simulink model "Subsistema_Fisico_No_Lineal"  (R2024b)
settings: Solver=VariableStepAuto  StartTime=0.0  StopTime=10.0  RelTol=1e-3
values from neighbouring files (symbols this model uses):
  alpha_cu = 3.9 *10^-3    (= 0.0039)    [parametros.m]
  b_eq = b_m + (1/r^2) * b_l    (= 2.19444444444e-05)    [parametros.m]
  C_ts = 0.818    [parametros.m]
  g = 9.80665    [parametros.m]
  J_eq = J_m + (1/r^2) * J_l    (= 4.58263888889e-05)    [parametros.m]
  k_l = m * l_cm + m_l* l_l    (= 1)    [parametros.m]
  L_d = 6.6 * 10^-3    (= 0.0066)    [parametros.m]
  L_ls = 0.8 * 10^-3    (= 0.0008)    [parametros.m]
  L_q = 5.8 * 10^-3    (= 0.0058)    [parametros.m]
  lambda_m = 0.016    [parametros.m]
  P_p = 3    [parametros.m]
  r = 120    [parametros.m]
  R_s_40 = 1.02    [parametros.m]
  R_ts_amb = 146.7    [parametros.m]
  Temp_s_ref = 20    [parametros.m]
settings Model: Creator=nsorr  LastModifiedBy=nsorr

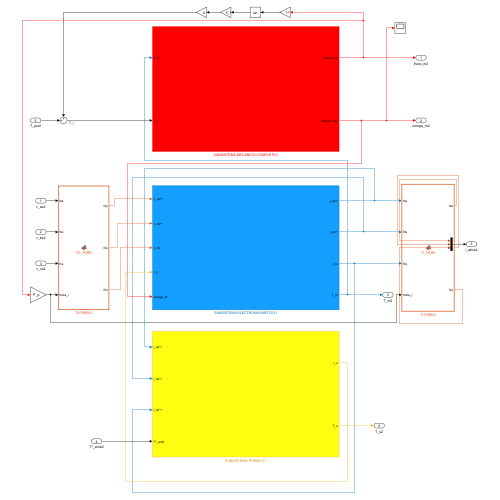
[thumbnail: Simulink's stored preview of the top-level diagram]
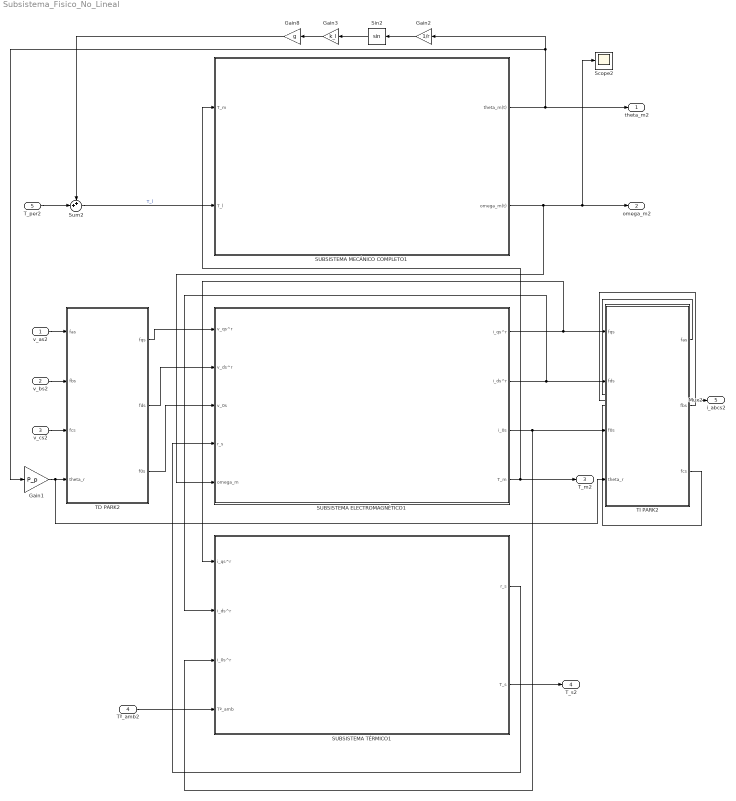
== system Subsistema_Fisico_No_Lineal ==
  v_as2 : Inport
  v_bs2 : Inport  Port=2
  v_cs2 : Inport  Port=3
  Tº_amb2 : Inport  Port=4
  T_per2 : Inport  Port=5
  Gain1 : Gain  Gain=P_p
  Gain2 : Gain  Gain=1/r
  Gain3 : Gain  Gain=k_l
  Gain8 : Gain  Gain=g
  Mux2 : Mux  Inputs=3
  SUBSISTEMA ELECTROMAGNÉTICO1 : Subsystem
  SUBSISTEMA MECÁNICO COMPLETO1 : Subsystem
  SUBSISTEMA TÉRMICO1 : Subsystem
  Scope2 : Scope
  Sin2 : Trigonometry
  Sum2 : Sum  Inputs=++|
  TD PARK2 : MATLAB Function  TreatAsAtomicUnit=on
  TI PARK2 : MATLAB Function  TreatAsAtomicUnit=on
  theta_m2 : Outport
  omega_m2 : Outport  Port=2
  T_m2 : Outport  Port=3
  T_s2 : Outport  Port=4
  i_abcs2 : Outport  Port=5
  wires:
  Sin2/1 -> Gain3/1
  Mux2/1 -> i_abcs2/1
  Gain3/1 -> Gain8/1
  TI PARK2/1(fas) -> Mux2/1
  v_cs2/1 -> TD PARK2/3(fcs)
  SUBSISTEMA ELECTROMAGNÉTICO1/2(i_ds^r) -> SUBSISTEMA TÉRMICO1/2(i_ds^r), TI PARK2/2(fds)
  Gain1/1 -> TI PARK2/4(theta_r), TD PARK2/4(theta_r)
  T_per2/1 -> Sum2/2
  SUBSISTEMA TÉRMICO1/1(r_s) -> SUBSISTEMA ELECTROMAGNÉTICO1/4(r_s)
  SUBSISTEMA ELECTROMAGNÉTICO1/1(i_qs^r) -> SUBSISTEMA TÉRMICO1/1(i_qs^r), TI PARK2/1(fqs)
  v_bs2/1 -> TD PARK2/2(fbs)
  Tº_amb2/1 -> SUBSISTEMA TÉRMICO1/4(Tº_amb)
  Gain2/1 -> Sin2/1
  SUBSISTEMA TÉRMICO1/2(T_s) -> T_s2/1
  TI PARK2/2(fbs) -> Mux2/2
  SUBSISTEMA ELECTROMAGNÉTICO1/4(T_m) -> SUBSISTEMA MECÁNICO COMPLETO1/1(T_m), T_m2/1
  SUBSISTEMA ELECTROMAGNÉTICO1/3(i_0s) -> SUBSISTEMA TÉRMICO1/3(i_0s^r), TI PARK2/3(f0s)
  TD PARK2/3(f0s) -> SUBSISTEMA ELECTROMAGNÉTICO1/3(v_0s)
  v_as2/1 -> TD PARK2/1(fas)
  Sum2/1 -> SUBSISTEMA MECÁNICO COMPLETO1/2(T_l)  "T_l"
  SUBSISTEMA MECÁNICO COMPLETO1/1(theta_m(t)) -> Gain2/1, Gain1/1, theta_m2/1
  TD PARK2/1(fqs) -> SUBSISTEMA ELECTROMAGNÉTICO1/1(v_qs^r)
  TI PARK2/3(fcs) -> Mux2/3
  SUBSISTEMA MECÁNICO COMPLETO1/2(omega_m(t)) -> SUBSISTEMA ELECTROMAGNÉTICO1/5(omega_m), omega_m2/1, Scope2/1
  Gain8/1 -> Sum2/1
  TD PARK2/2(fds) -> SUBSISTEMA ELECTROMAGNÉTICO1/2(v_ds^r)

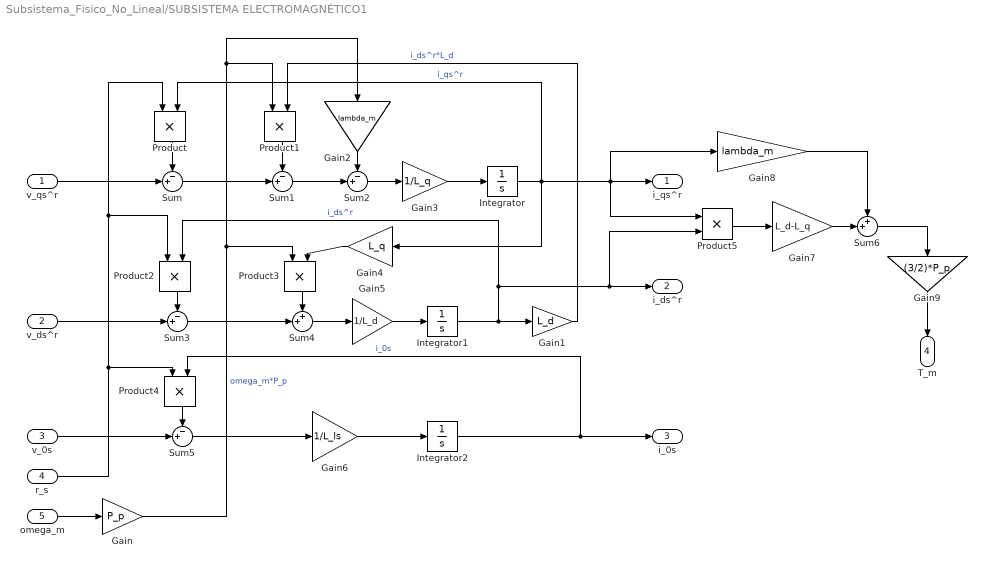
== system Subsistema_Fisico_No_Lineal/SUBSISTEMA ELECTROMAGNÉTICO1 ==
  v_qs^r : Inport
  v_ds^r : Inport  Port=2
  v_0s : Inport  Port=3
  r_s : Inport  Port=4
  omega_m : Inport  Port=5
  Gain : Gain  Gain=P_p
  Gain1 : Gain  Gain=L_d
  Gain2 : Gain  Gain=lambda_m
  Gain3 : Gain  Gain=1/L_q
  Gain4 : Gain  Gain=L_q
  Gain5 : Gain  Gain=1/L_d
  Gain6 : Gain  Gain=1/L_ls
  Gain7 : Gain  Gain=L_d-L_q
  Gain8 : Gain  Gain=lambda_m
  Gain9 : Gain  Gain=(3/2)*P_p
  Integrator : Integrator
  Integrator1 : Integrator
  Integrator2 : Integrator
  Product{,1..5} (6 alike) : Product
  Sum{,1..3,5} (5 alike) : Sum  Inputs=-+|
  Sum4 : Sum  Inputs=++|
  Sum6 : Sum  Inputs=++|
  i_qs^r : Outport
  i_ds^r : Outport  Port=2
  i_0s : Outport  Port=3
  T_m : Outport  Port=4
  wires:
  v_ds^r/1 -> Sum3/2
  Gain2/1 -> Sum2/1
  Sum6/1 -> Gain9/1
  Product/1 -> Sum/1
  v_qs^r/1 -> Sum/2
  Sum/1 -> Sum1/2
  Gain7/1 -> Sum6/2
  omega_m/1 -> Gain/1
  Gain/1 -> Gain2/1, Product1/1, Product3/1  "omega_m*P_p"
  Integrator2/1 -> i_0s/1, Product4/2  "i_0s"
  Product5/1 -> Gain7/1
  Integrator1/1 -> Product2/2, i_ds^r/1, Product5/2, Gain1/1  "i_ds^r"
  Gain8/1 -> Sum6/1
  Product3/1 -> Sum4/1
  v_0s/1 -> Sum5/2
  Gain9/1 -> T_m/1
  Gain3/1 -> Integrator/1
  Sum2/1 -> Gain3/1
  Integrator/1 -> i_qs^r/1, Gain8/1, Product5/1, Product/2, Gain4/1  "i_qs^r"
  r_s/1 -> Product4/1, Product/1, Product2/1
  Sum4/1 -> Gain5/1
  Sum1/1 -> Sum2/2
  Gain5/1 -> Integrator1/1
  Gain4/1 -> Product3/2
  Sum3/1 -> Sum4/2
  Product4/1 -> Sum5/1
  Product2/1 -> Sum3/1
  Gain1/1 -> Product1/2  "i_ds^r*L_d"
  Gain6/1 -> Integrator2/1
  Sum5/1 -> Gain6/1
  Product1/1 -> Sum1/1

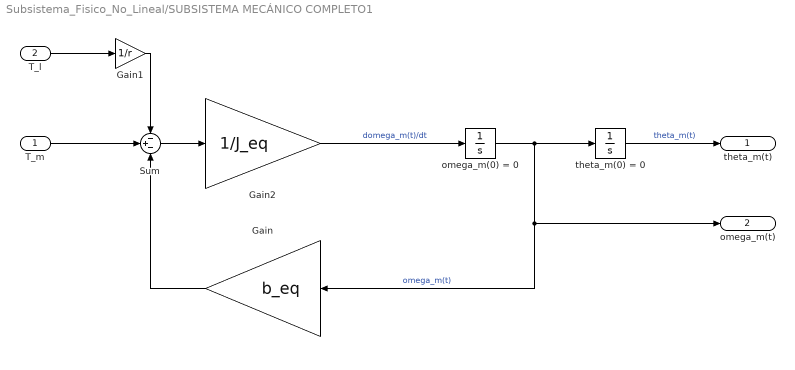
== system Subsistema_Fisico_No_Lineal/SUBSISTEMA MECÁNICO COMPLETO1 ==
  T_m : Inport
  T_l : Inport  Port=2
  Gain : Gain  Gain=b_eq
  Gain1 : Gain  Gain=1/r
  Gain2 : Gain  Gain=1/J_eq
  Sum : Sum  Inputs=-+-
  omega_m(0) = 0 : Integrator
  theta_m(0) = 0 : Integrator
  theta_m(t) : Outport
  omega_m(t) : Outport  Port=2
  wires:
  omega_m(0) = 0/1 -> omega_m(t)/1, Gain/1, theta_m(0) = 0/1  "omega_m(t)"
  T_m/1 -> Sum/2
  Gain2/1 -> omega_m(0) = 0/1  "domega_m(t)/dt"
  Sum/1 -> Gain2/1
  Gain/1 -> Sum/3
  Gain1/1 -> Sum/1
  T_l/1 -> Gain1/1
  theta_m(0) = 0/1 -> theta_m(t)/1  "theta_m(t)"

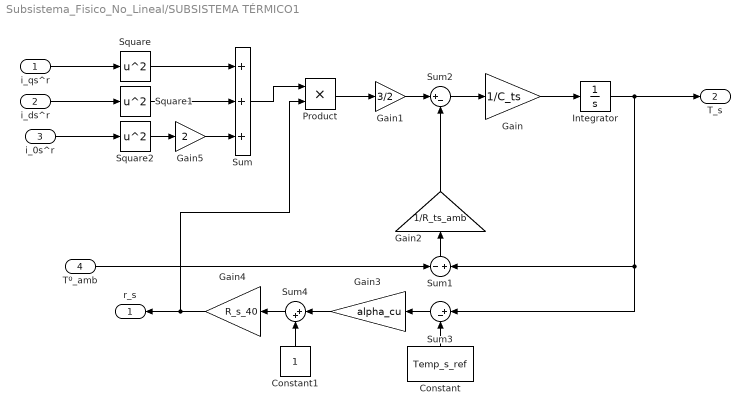
== system Subsistema_Fisico_No_Lineal/SUBSISTEMA TÉRMICO1 ==
  i_qs^r : Inport
  i_ds^r : Inport  Port=2
  i_0s^r : Inport  Port=3
  Tº_amb : Inport  Port=4
  Constant : Constant  Value=Temp_s_ref
  Constant1 : Constant
  Gain : Gain  Gain=1/C_ts
  Gain1 : Gain  Gain=3/2
  Gain2 : Gain  Gain=1/R_ts_amb
  Gain3 : Gain  Gain=alpha_cu
  Gain4 : Gain  Gain=R_s_40
  Gain5 : Gain  Gain=2
  Integrator : Integrator  InitialCondition=40
  Product : Product
  Square : Math  Operator=square
  Square1 : Math  Operator=square
  Square2 : Math  Operator=square
  Sum : Sum  Inputs=+++
  Sum1 : Sum  Inputs=-|+
  Sum2 : Sum  Inputs=|+-
  Sum3 : Sum  Inputs=|+-
  Sum4 : Sum  Inputs=|++
  r_s : Outport
  T_s : Outport  Port=2
  wires:
  Gain4/1 -> r_s/1, Product/2
  Gain/1 -> Integrator/1
  Square/1 -> Sum/1
  i_0s^r/1 -> Square2/1
  Gain1/1 -> Sum2/1
  Sum/1 -> Product/1
  Gain3/1 -> Sum4/1
  Gain5/1 -> Sum/3
  Sum4/1 -> Gain4/1
  Gain2/1 -> Sum2/2
  Square1/1 -> Sum/2
  Constant1/1 -> Sum4/2
  Tº_amb/1 -> Sum1/1
  i_ds^r/1 -> Square1/1
  i_qs^r/1 -> Square/1
  Constant/1 -> Sum3/2
  Sum1/1 -> Gain2/1
  Sum3/1 -> Gain3/1
  Product/1 -> Gain1/1
  Integrator/1 -> T_s/1, Sum3/1, Sum1/2
  Sum2/1 -> Gain/1
  Square2/1 -> Gain5/1

== matlab function Subsistema_Fisico_No_Lineal/TD PARK2 ==
  data: fas input; fqs output; fbs input; fcs input; theta_r input; fds output; f0s output
function [fqs, fds, f0s] = TD_PARK(fas, fbs, fcs, theta_r)

    fabcs = [fas; fbs; fcs];

    Ks = 2/3*[cos(theta_r) cos(theta_r - 2*pi/3) cos(theta_r + 2*pi/3)
          sin(theta_r) sin(theta_r - 2*pi/3) sin(theta_r + 2*pi/3) 
          1/2          1/2                   1/2];

    fqd0s = Ks * fabcs;

    fqs = fqd0s(1);
    fds = fqd0s(2);
    f0s = fqd0s(3);

end

== matlab function Subsistema_Fisico_No_Lineal/TI PARK2 ==
  data: fqs input; fas output; fds input; f0s input; theta_r input; fbs output; fcs output
function [fas, fbs, fcs] = TI_PARK(fqs, fds, f0s , theta_r)

    fqd0s = [fqs; fds; f0s];

    Ks = [cos(theta_r)         sin(theta_r)             1
          cos(theta_r - 2*pi/3) sin(theta_r - 2*pi/3)    1
          cos(theta_r + 2*pi/3) sin(theta_r + 2*pi/3)    1];

    fabcs = Ks * fqd0s;

    fas = fabcs(1);
    fbs = fabcs(2);
    fcs = fabcs(3);

end
